simulink model "minseg_M2V3_2017a"  (R2017a)
settings: Solver=FixedStepDiscrete  StartTime=0.0  StopTime=inf  FixedStep=mdl_T_sample  RelTol=1e-3
undefined symbols (not defined in the file or in its folder): ctrl_lqr_K2, ctrl_motorDriver_v_ff_cmd_v_val, ctrl_motorDriver_v_ff_cmd_v_val_norm_dx_max, ctrl_motorDriver_v_ff_cmd_v_val_norm_dx_min, ctrl_motorDriver_v_output_max, ctrl_motorDriver_v_output_min, ctrl_motorDriver_v_pid_cmd_thetaDot_val, ctrl_motorDriver_v_pid_cmd_thetaDot_val_norm_dx_max, ctrl_motorDriver_v_pid_cmd_thetaDot_val_norm_dx_min, ctrl_motorDriver_v_pid_int_maxVal, ctrl_motorDriver_v_pid_int_minVal, ctrl_motorDriver_v_pid_k_d, ctrl_motorDriver_v_pid_k_i, ctrl_motorDriver_v_pid_k_p, ctrl_motorDriver_v_rts_ss_k_A, ctrl_motorDriver_v_rts_ss_k_B, ctrl_motorDriver_v_rts_ss_k_C, ctrl_motorDriver_v_rts_ss_k_D, ctrl_motorDriver_v_rts_ss_stateIC, ctrl_motorDriver_v_sfr_cmd_p_x_f, ctrl_motorDriver_v_sfr_cmd_p_x_mag, ctrl_motorDriver_v_sfr_cmd_p_y_f, ctrl_motorDriver_v_sfr_cmd_p_y_mag, ctrl_motorDriver_v_sfr_K, ctrl_motorDriver_v_sfr_K_plant, ctrl_motorDriver_v_sfr_K_rts, ctrl_motorDriver_v_T_cmd, ctrl_motorDriver_v_T_init, DiscIntNeverNeededParam, gyro_bias, io_srl_read_rateTransition_initialCondition, k_intmax_uint8, mdl_T_sample, mtr_encoder_filter_z_ss_A, mtr_encoder_filter_z_ss_B, mtr_encoder_filter_z_ss_C, mtr_encoder_filter_z_ss_D, plant, plant_accel_k_digital2analog, plant_body_l_c, plant_body_l_w, plant_gyro_encoder_filter_z_den, plant_gyro_encoder_filter_z_num, plant_gyro_filter_z_den, plant_gyro_filter_z_num, plant_gyro_k_digital2analog, plant_linear_ss_stateIC, plant_linear_ss_t_A, plant_linear_ss_t_B, plant_linear_ss_t_C, plant_linear_ss_t_D, plant_mtr_encoder_count2wheelRad, plant_mtr_encoder_filter_z_den, plant_mtr_encoder_filter_z_num, plant_pSupply_v, plant_supply_v, plant_T_init, plant_wheel_r
undefined symbols (not defined in the file): ctrl_lqr_addlDyn_A_discrete, ctrl_lqr_addlDyn_B_discrete, ctrl_lqr_addlDyn_C_discrete, ctrl_lqr_addlDyn_D_discrete, ctrl_lqr_addlDyn_k_antiWindup, ctrl_lqr_addlDyn_stateIC, plant_gyro_bias_movingAverage_n_pts, plant_linear_A_continuous, plant_linear_B_continuous, plant_linear_C_continuous, plant_linear_D_continuous, plant_linear_stateIC
libraries: svdutilitieslib x135, simulink x57, arduinolib x15, MinSegLibrary_M2V3 x3, dspindex x3, RASPlib x2
(part 2 of 6)

== system minseg_M2V3_2017a/Controller [v.motorDriver]/Controller and Enable/Controller/State Feedback Regulation with Reference Tracking System ==
  userIO.read.controller.command : Inport
  plant.state : Inport  Port=2
  Add : Sum  Inputs=-+
  Add1 : Sum  Inputs=--
  Additional Dynamics for Reference Tracking System [Discrete State-Space] : DiscreteStateSpace  A=ctrl_motorDriver_v_rts_ss_k_A  B=ctrl_motorDriver_v_rts_ss_k_B  C=ctrl_motorDriver_v_rts_ss_k_C  D=ctrl_motorDriver_v_rts_ss_k_D  X0=ctrl_motorDriver_v_rts_ss_stateIC  SampleTime=-1
  Gain : Gain  Gain=ctrl_motorDriver_v_sfr_K_plant  Multiplication=Matrix(K*u)
      settings: AttributesFormatString=%<Gain>
  Gain1 : Gain  Gain=ctrl_motorDriver_v_sfr_K_rts  Multiplication=Matrix(K*u)
      settings: AttributesFormatString=%<Gain>
  bus2mux [Command: Reference Tracking System] : Subsystem
  bus2mux [State: Plant] : Subsystem
  bus2mux [State: Reference Tracking System] : Subsystem
  mux2bus [Error: Reference Tracking System] : Subsystem
  output : Outport
  error : Outport  Port=2
  wires:
  bus2mux [State: Reference Tracking System]/1(mux) -> Add/2  "state"
  [KpXp] -> Add1/1  "plant"
  Add/1 -> mux2bus [Error: Reference Tracking System]/1(mux), Additional Dynamics for Reference Tracking System [Discrete State-Space]/1  "error"
  bus2mux [State: Plant]/1(mux) -> Gain/1  "state"
  [plant_state] -> bus2mux [State: Plant]/1(bus)
  plant.state/1 -> [plant_state]
  Additional Dynamics for Reference Tracking System [Discrete State-Space]/1 -> Gain1/1
  Gain1/1 -> Add1/2  "referenceTrackingSystem"
  bus2mux [Command: Reference Tracking System]/1(mux) -> Add/1  "reference"
  Add1/1 -> output/1
  userIO.read.controller.command/1 -> bus2mux [Command: Reference Tracking System]/1(bus)
  Gain/1 -> [KpXp]
  [plant_state] -> bus2mux [State: Reference Tracking System]/1(bus)
  mux2bus [Error: Reference Tracking System]/1(bus) -> error/1

== system minseg_M2V3_2017a/Controller [v.motorDriver]/Saturation/Left-Connected Motor/Saturation flag ==
  u.max : Inport
  u.raw : Inport  Port=2
  u.min : Inport  Port=3
  Add : Sum
  Data Type Conversion : DataTypeConversion  OutDataTypeStr=uint8
  Data Type Conversion1 : DataTypeConversion  OutDataTypeStr=uint8
  Gain : Gain  Gain=uint8(2)  OutDataTypeStr=uint8
      settings: AttributesFormatString=%<Gain>
  Gain1 : Gain  Gain=uint8(1)  OutDataTypeStr=uint8
      settings: AttributesFormatString=%<Gain>
  Relational Operator : RelationalOperator  OutDataTypeStr=boolean  RndMeth=Nearest
  Relational Operator1 : RelationalOperator  Operator=<=  OutDataTypeStr=boolean  RndMeth=Nearest
  x.saturating : Outport
  wires:
  u.raw/1 -> [u_raw]
  [u_raw] -> Relational Operator/1
  u.max/1 -> Relational Operator/2
  [u_raw] -> Relational Operator1/1
  u.min/1 -> Relational Operator1/2
  Add/1 -> x.saturating/1  "x.saturating"
  Relational Operator1/1 -> Data Type Conversion1/1  "x.lowerSaturating"
  Relational Operator/1 -> Data Type Conversion/1  "x.upperSaturating"
  Data Type Conversion/1 -> Gain/1
  Data Type Conversion1/1 -> Gain1/1
  Gain/1 -> Add/1
  Gain1/1 -> Add/2

== system minseg_M2V3_2017a/Controller [v.motorDriver]/Saturation/Middle-Connected Motor/Saturation flag ==
  u.max : Inport
  u.raw : Inport  Port=2
  u.min : Inport  Port=3
  Add : Sum
  Data Type Conversion : DataTypeConversion  OutDataTypeStr=uint8
  Data Type Conversion1 : DataTypeConversion  OutDataTypeStr=uint8
  Gain : Gain  Gain=uint8(2)  OutDataTypeStr=uint8
      settings: AttributesFormatString=%<Gain>
  Gain1 : Gain  Gain=uint8(1)  OutDataTypeStr=uint8
      settings: AttributesFormatString=%<Gain>
  Relational Operator : RelationalOperator  OutDataTypeStr=boolean  RndMeth=Nearest
  Relational Operator1 : RelationalOperator  Operator=<=  OutDataTypeStr=boolean  RndMeth=Nearest
  x.saturating : Outport
  wires:
  Gain1/1 -> Add/2
  Gain/1 -> Add/1
  Data Type Conversion1/1 -> Gain1/1
  Data Type Conversion/1 -> Gain/1
  Relational Operator/1 -> Data Type Conversion/1  "x.upperSaturating"
  Relational Operator1/1 -> Data Type Conversion1/1  "x.lowerSaturating"
  Add/1 -> x.saturating/1  "x.saturating"
  u.min/1 -> Relational Operator1/2
  [u_raw] -> Relational Operator1/1
  u.max/1 -> Relational Operator/2
  [u_raw] -> Relational Operator/1
  u.raw/1 -> [u_raw]

== system minseg_M2V3_2017a/Plant/Hardware/Analog to Digital Conversion/Motor Driver ==
  left.voltage.command : Inport
  middle.voltage.command : Inport  Port=2
  Bus Creator : BusCreator  Inputs=2
  Bus Creator1 : BusCreator  Inputs=2
  Bus Creator{2..4,6,8..9} (6 alike) : BusCreator  Inputs=1
  Left-Connected : Subsystem
  Middle-Connected : Subsystem
  left : Outport
  middle : Outport  Port=2
  wires:
  Bus Creator1/1 -> Bus Creator4/1  "digital"
  Middle-Connected/1(voltage.command.digital.positive) -> Bus Creator1/1  "positive [V]"
  Middle-Connected/2(voltage.command.digital.negative) -> Bus Creator1/2  "negative [V]"
  Bus Creator2/1 -> Bus Creator3/1  "voltage"
  Bus Creator3/1 -> middle/1
  Bus Creator4/1 -> Bus Creator2/1  "command"
  Bus Creator9/1 -> Bus Creator6/1  "command"
  Bus Creator8/1 -> left/1
  middle.voltage.command/1 -> Middle-Connected/1(voltage.command.analog)
  left.voltage.command/1 -> Left-Connected/1(voltage.command.analog)
  Bus Creator6/1 -> Bus Creator8/1  "voltage"
  Left-Connected/2(voltage.command.digital.negative) -> Bus Creator/2  "negative [V]"
  Left-Connected/1(voltage.command.digital.positive) -> Bus Creator/1  "positive [V]"
  Bus Creator/1 -> Bus Creator9/1  "digital"

== system minseg_M2V3_2017a/Plant/Hardware/Arduino Pin IO/Digital Inputs (Reads from Pins) ==
  Accelerometer soMPU6050 : MATLABSystem  System=soMPU6050Accel  SimulateUsing=Code generation
      mask Type: soMPU6050Accel
      mask Display:
      | disp('soMPU6050Accel');
      | port_label('output',1,'xaccel');
      | port_label('output',2,'yaccel');
      | port_label('output',3,'zaccel');
  Bus Creator{1..5,7..8,10..13,16..17} (13 alike) : BusCreator  Inputs=1
  Bus Creator14 : BusCreator  Inputs=2
  Bus Creator15 : BusCreator  Inputs=3
  Bus Creator6 : BusCreator  Inputs=3
  Bus Creator9 : BusCreator  Inputs=3
  Encoder M2V3 - Left Connected - Pins 19,18 : MinSegLibrary_M2V3/M2V3 Left Connector 18, 19  Encoder=1  PinA=19  PinB=18  PWMFSelect=3  PWMTimer=-1
      settings: SourceProductName=Rensselaer Arduino Support Package
  "Encoder M2V3 - Middle Connected - Pins 62, 15" : MinSegLibrary_M2V3/M2V3 Middle Connector 15, 62  Encoder=3  PinA=15  PinB=62  PWMFSelect=3  PWMTimer=-1
      settings: SourceProductName=Rensselaer Arduino Support Package
  Gyroscope soMPU6050 : RASPlib/Gyroscope  DLPFmode=plant_gyro_dlpf_mode
      settings: AttributesFormatString=DLPF mode: %<DLPFmode>  SourceProductName=Rensselaer Arduino Support Package
  Magnetometer : MATLABSystem  System=soHMC5883L  SimulateUsing=Code generation
      mask Type: soHMC5883L
      mask Display:
      | disp('soHMC5883L');
      | port_label('output',1,'xmag');
      | port_label('output',2,'ymag');
      | port_label('output',3,'zmag');
  Pushbutton - Pin A3 : MinSegLibrary_M2V3/User Pushbutton A3  Pin=3
      settings: SourceProductName=Rensselaer Arduino Support Package
  Temperature Sensor (Unspecified) : RASPlib/Temperature  SimulateUsing=Code generation
      settings: SourceProductName=Rensselaer Arduino Support Package
  gyroscope : Outport
  accelerometer : Outport  Port=2
  motorEncoder : Outport  Port=3
  magnetometer : Outport  Port=4
  pushbutton : Outport  Port=5
  tempometer : Outport  Port=6
  wires:
  Bus Creator5/1 -> Bus Creator9/1  "x"
  Bus Creator11/1 -> Bus Creator9/3  "z"
  Encoder M2V3 - Left Connected - Pins 19,18/1 -> Bus Creator13/1  "digital [-]"
  Bus Creator2/1 -> Bus Creator14/2  "middle"
  Bus Creator10/1 -> Bus Creator9/2  "y"
  "Encoder M2V3 - Middle Connected - Pins 62, 15"/1 -> Bus Creator2/1  "digital [-]"
  Accelerometer soMPU6050/3 -> Bus Creator11/1  "digital [-]"
  Accelerometer soMPU6050/1 -> Bus Creator5/1  "digital [-]"
  Accelerometer soMPU6050/2 -> Bus Creator10/1  "digital [-]"
  Bus Creator9/1 -> accelerometer/1
  Bus Creator14/1 -> motorEncoder/1
  Bus Creator13/1 -> Bus Creator14/1  "left"
  Bus Creator3/1 -> Bus Creator6/1  "x"
  Gyroscope soMPU6050/2 -> Bus Creator7/1  "digital [-]"
  Bus Creator6/1 -> gyroscope/1
  Gyroscope soMPU6050/3 -> Bus Creator8/1  "digital [-]"
  Bus Creator7/1 -> Bus Creator6/2  "y"
  Gyroscope soMPU6050/1 -> Bus Creator3/1  "digital [-]"
  Bus Creator8/1 -> Bus Creator6/3  "z"
  Bus Creator15/1 -> magnetometer/1
  Magnetometer/2 -> Bus Creator1/1  "digital [-]"
  Magnetometer/1 -> Bus Creator12/1  "digital [-]"
  Magnetometer/3 -> Bus Creator4/1  "digital [-]"
  Bus Creator1/1 -> Bus Creator15/2  "y"
  Bus Creator4/1 -> Bus Creator15/3  "z"
  Bus Creator12/1 -> Bus Creator15/1  "x"
  Pushbutton - Pin A3/1 -> Bus Creator16/1  "digital [-]"
  Bus Creator16/1 -> pushbutton/1
  Temperature Sensor (Unspecified)/1 -> Bus Creator17/1  "digital [-]"
  Bus Creator17/1 -> tempometer/1

== system minseg_M2V3_2017a/Plant/Hardware/Arduino Pin IO/Digital Outputs (Writes to Pins) ==
  motorDriver.left.voltage.command.digital.positive : Inport
  motorDriver.left.voltage.command.digital.negative : Inport  Port=2
  motorDriver.middle.voltage.command.digital.positive : Inport  Port=3
  motorDriver.middle.voltage.command.digital.negative : Inport  Port=4
  Motor : Subsystem
  wires:
  motorDriver.left.voltage.command.digital.positive/1 -> Motor/1(motor.left.voltage.command.digital.positive)
  motorDriver.left.voltage.command.digital.negative/1 -> Motor/2(motor.left.voltage.command.digital.negative)
  motorDriver.middle.voltage.command.digital.positive/1 -> Motor/3(motor.middle.voltage.command.digital.positive)
  motorDriver.middle.voltage.command.digital.negative/1 -> Motor/4(motor.middle.voltage.command.digital.negative)

== system minseg_M2V3_2017a/Plant/Hardware/Calculations/Body Angular Position (phi) ==
  gyroscope.x : Inport
  gyroscope.y : Inport  Port=2
  gyroscope.z : Inport  Port=3
  accelerometer.x : Inport  Port=4
  accelerometer.y : Inport  Port=5
  accelerometer.z : Inport  Port=6
  wheel.angularPosition.global.left : Inport  Port=7
  wheel.angularPosition.global.middle : Inport  Port=8
  clock.timedEvent.plant.x_initialization : Inport  Port=9
  Bus Creator : BusCreator  Inputs=2
  Bus Creator1 : BusCreator  Inputs=2
  Bus Creator2 : BusCreator  Inputs=2
  X (Pitch) : Subsystem  Variant=on  VariantControl=Variant1
  Y (Yaw) : Subsystem  Variant=on  VariantControl=Variant1
  Z (Roll) : Subsystem  Variant=on  VariantControl=Variant1
  x : Outport
  y : Outport  Port=2
  z : Outport  Port=3
  wires:
  Bus Creator1/1 -> y/1
  Bus Creator/1 -> x/1
  Y (Yaw)/1(" position.y") -> Bus Creator1/1  "position [rad]"
  X (Pitch)/1(" position.x") -> Bus Creator/1  "position [rad]"
  X (Pitch)/2(velocity.x) -> Bus Creator/2  "velocity [rad/s]"
  Z (Roll)/1(position.z) -> Bus Creator2/1  "position [rad]"
  Bus Creator2/1 -> z/1
  gyroscope.x/1 -> X (Pitch)/1(gyroscope.x)
  gyroscope.y/1 -> Y (Yaw)/1(gyroscope.y)
  gyroscope.z/1 -> Z (Roll)/1(gyroscope.z)
  wheel.angularPosition.global.left/1 -> Y (Yaw)/2(wheel.angularPosition.global.left)
  wheel.angularPosition.global.middle/1 -> Y (Yaw)/3(wheel.angularPosition.global.middle)
  accelerometer.y/1 -> [accel_y]
  [accel_y] -> X (Pitch)/2(accelerometer.y)
  accelerometer.z/1 -> [accel_z]
  [accel_z] -> X (Pitch)/3(accelerometer.z)
  Y (Yaw)/2(velocity.y) -> Bus Creator1/2  "velocity [rad/s]"
  Z (Roll)/2(velocity.z) -> Bus Creator2/2  "velocity [rad/s]"
  [accel_y] -> Z (Roll)/3(accelerometer.y)
  [accel_z] -> Z (Roll)/4(accelerometer.z)
  accelerometer.x/1 -> Z (Roll)/2(accelerometer.x)
  clock.timedEvent.plant.x_initialization/1 -> [x_init]
  [x_init] -> X (Pitch)/4(clock.timedEvent.plant.x_initialization)
  [x_init] -> Y (Yaw)/4(clock.timedEvent.plant.x_initialization)
  [x_init] -> Z (Roll)/5(clock.timedEvent.plant.x_initialization)

== system minseg_M2V3_2017a/Plant/Hardware/Calculations/Linear Position (p) ==
  wheel.angularVelocity.global : Inport
  body.angularPosition.x (pitch) : Inport  Port=2
  body.angularPosition.y (yaw) : Inport  Port=3
  Body : Subsystem
  Bus Creator1 : BusCreator  Inputs=3
  Bus Creator4 : BusCreator  Inputs=3
  Bus Selector1 : BusSelector  OutputSignals=center.x.position [m],center.y.position [m],center.z.position [m]
  Wheel : Subsystem
  wheel : Outport
  body : Outport  Port=2
  wires:
  [p_wheel] -> Bus Selector1/1
  Bus Creator4/1 -> [p_wheel], wheel/1
  Wheel/3(center) -> Bus Creator4/3  "center"
  wheel.angularVelocity.global/1 -> Wheel/1(wheel.angularVelocity.global)
  Wheel/2(middle) -> Bus Creator4/2  "middle"
  Wheel/1(left) -> Bus Creator4/1  "left"
  Bus Selector1/2 -> Body/2(p.center.y)  "<position [m]>"
  Bus Selector1/1 -> Body/1(p.center.x)  "<position [m]>"
  Bus Selector1/3 -> Body/3(p.center.z)  "<position [m]>"
  body.angularPosition.y (yaw)/1 -> [yaw]
  [yaw] -> Wheel/2(body.angularPosition.y (yaw))
  body.angularPosition.x (pitch)/1 -> Body/4(body.angularPosition.x (pitch))
  [yaw] -> Body/5(body.angularPosition.y (yaw))
  Bus Creator1/1 -> body/1
  Body/1(x) -> Bus Creator1/1  "x"
  Body/2(y) -> Bus Creator1/2  "y"
  Body/3(z) -> Bus Creator1/3  "z"

== system minseg_M2V3_2017a/Plant/Hardware/Calculations/Wheel Angular Position (theta) ==
  motorEncoder.left : Inport
  motorEncoder.middle : Inport  Port=2
  body.angularPosition.x (pitch) : Inport  Port=3
  Bus Creator1 : BusCreator  Inputs=3
  Bus Creator4 : BusCreator  Inputs=3
  Bus Selector1 : BusSelector  OutputSignals=left.position [rad],middle.position [rad]
  Reference Point: Body : Subsystem
  Reference Point: Earth : Subsystem
  body : Outport
  global : Outport  Port=2
  wires:
  motorEncoder.left/1 -> Reference Point: Body/1(motorEncoder.left)
  motorEncoder.middle/1 -> Reference Point: Body/2(motorEncoder.middle)
  Bus Creator4/1 -> [theta_body], body/1
  Bus Creator1/1 -> global/1
  Reference Point: Body/2(middle) -> Bus Creator4/2  "middle"
  Reference Point: Body/1(left) -> Bus Creator4/1  "left"
  Reference Point: Body/3(average) -> Bus Creator4/3  "average"
  [theta_body] -> Bus Selector1/1
  Reference Point: Earth/1(left) -> Bus Creator1/1  "left"
  Reference Point: Earth/2(middle) -> Bus Creator1/2  "middle"
  Reference Point: Earth/3(average) -> Bus Creator1/3  "average"
  Bus Selector1/1 -> Reference Point: Earth/1(wheel.left.angularPosition.body)  "<position [rad]>"
  Bus Selector1/2 -> Reference Point: Earth/2(wheel.middle.angularPosition.body)  "<position [rad]>"
  body.angularPosition.x (pitch)/1 -> Reference Point: Earth/3(body.angularPosition.x (pitch))

== system minseg_M2V3_2017a/Plant/Hardware/Digital to Analog Conversion/Accelerometer ==
  x.digital : Inport
  y.digital : Inport  Port=2
  z.digital : Inport  Port=3
  Data Type Conversion1 : DataTypeConversion  OutDataTypeStr=double
  Data Type Conversion2 : DataTypeConversion  OutDataTypeStr=double
  Data Type Conversion3 : DataTypeConversion  OutDataTypeStr=double
  Gain1 : Gain  Gain=plant_accel_k_digital2analog
      settings: AttributesFormatString=%<Gain>
  Gain2 : Gain  Gain=plant_accel_k_digital2analog
      settings: AttributesFormatString=%<Gain>
  Gain3 : Gain  Gain=plant_accel_k_digital2analog
      settings: AttributesFormatString=%<Gain>
  x.analog : Outport
  y.analog : Outport  Port=2
  z.analog : Outport  Port=3
  wires:
  z.digital/1 -> Data Type Conversion3/1
  y.digital/1 -> Data Type Conversion2/1
  Gain2/1 -> y.analog/1
  Gain3/1 -> z.analog/1
  Gain1/1 -> x.analog/1
  Data Type Conversion1/1 -> Gain1/1
  x.digital/1 -> Data Type Conversion1/1
  Data Type Conversion2/1 -> Gain2/1
  Data Type Conversion3/1 -> Gain3/1

== system minseg_M2V3_2017a/Plant/Hardware/Digital to Analog Conversion/Gyroscope ==
  x.digital : Inport
  y.digital : Inport  Port=2
  z.digital : Inport  Port=3
  clock.timedEvent.plant.x_initialization : Inport  Port=4
  x : Subsystem
  y : Subsystem
  z : Subsystem
  x.analog : Outport
  y.analog : Outport  Port=2
  z.analog : Outport  Port=3
  wires:
  x/1(analog) -> x.analog/1
  x.digital/1 -> x/1(digital)
  [x_init] -> x/2(clock.timedEvent.plant.x_initialization)
  clock.timedEvent.plant.x_initialization/1 -> [x_init]
  [x_init] -> y/2(clock.timedEvent.model.initialization)
  y.digital/1 -> y/1(digital)
  y/1(analog) -> y.analog/1
  [x_init] -> z/2(clock.timedEvent.model.initialization)
  z.digital/1 -> z/1(digital)
  z/1(analog) -> z.analog/1

== system minseg_M2V3_2017a/Plant/Hardware/Digital to Analog Conversion/Magnetometer (Incomplete) ==
  x.digital : Inport
  y.digital : Inport  Port=2
  z.digital : Inport  Port=3
  Data Type Conversion1 : DataTypeConversion  OutDataTypeStr=double
  Data Type Conversion2 : DataTypeConversion  OutDataTypeStr=double
  Data Type Conversion3 : DataTypeConversion  OutDataTypeStr=double
  x.analog : Outport
  y.analog : Outport  Port=2
  z.analog : Outport  Port=3
  wires:
  y.digital/1 -> Data Type Conversion2/1
  z.digital/1 -> Data Type Conversion3/1
  x.digital/1 -> Data Type Conversion1/1
  Data Type Conversion1/1 -> x.analog/1
  Data Type Conversion2/1 -> y.analog/1
  Data Type Conversion3/1 -> z.analog/1

== system minseg_M2V3_2017a/Plant/Hardware/Digital to Analog Conversion/Motor Encoder ==
  left.digital : Inport
  middle.digital : Inport  Port=2
  Data Type Conversion : DataTypeConversion  OutDataTypeStr=double
      settings: AttributesFormatString=saturateOverflow(%<SaturateOnIntegerOverflow>)
  Data Type Conversion1 : DataTypeConversion  OutDataTypeStr=double
      settings: AttributesFormatString=saturateOverflow(%<SaturateOnIntegerOverflow>)
  Gain3 : Gain  Gain=plant_mtr_encoder_count2wheelRad
      settings: AttributesFormatString=%<Gain>
  Gain4 : Gain  Gain=plant_mtr_encoder_count2wheelRad
      settings: AttributesFormatString=%<Gain>
  left.analog : Outport
  middle.analog : Outport  Port=2
  wires:
  middle.digital/1 -> Data Type Conversion1/1
  left.digital/1 -> Data Type Conversion/1
  Data Type Conversion/1 -> Gain4/1
  Data Type Conversion1/1 -> Gain3/1
  Gain4/1 -> left.analog/1
  Gain3/1 -> middle.analog/1

== system minseg_M2V3_2017a/Plant/Hardware/Digital to Analog Conversion/Pushbutton (Incomplete) ==
  digital : Inport
  Data Type Conversion1 : DataTypeConversion  OutDataTypeStr=double
  analog : Outport
  wires:
  digital/1 -> Data Type Conversion1/1
  Data Type Conversion1/1 -> analog/1

== system minseg_M2V3_2017a/Plant/Hardware/Digital to Analog Conversion/Tempometer (Incomplete) ==
  digital : Inport
  Data Type Conversion1 : DataTypeConversion  OutDataTypeStr=double
  analog : Outport
  wires:
  digital/1 -> Data Type Conversion1/1
  Data Type Conversion1/1 -> analog/1

== system minseg_M2V3_2017a/Plant/Hardware-Equivalent Linear Dynamics/Calculation/Linear Position (p) ==
  wheel.angularVelocity.global : Inport
  body.angularPosition.x (pitch) : Inport  Port=2
  body.angularPosition.y (yaw) : Inport  Port=3
  Body : Subsystem
  Bus Creator1 : BusCreator  Inputs=3
  Bus Creator4 : BusCreator  Inputs=3
  Bus Selector1 : BusSelector  OutputSignals=center.x.position [m],center.y.position [m],center.z.position [m]
  Wheel : Subsystem
  wheel : Outport
  body : Outport  Port=2
  wires:
  [p_wheel] -> Bus Selector1/1
  Bus Creator4/1 -> [p_wheel], wheel/1
  Wheel/3(center) -> Bus Creator4/3  "center"
  wheel.angularVelocity.global/1 -> Wheel/1(wheel.angularVelocity.global)
  Wheel/2(middle) -> Bus Creator4/2  "middle"
  Wheel/1(left) -> Bus Creator4/1  "left"
  Bus Selector1/2 -> Body/2(p.center.y)  "<position [m]>"
  Bus Selector1/1 -> Body/1(p.center.x)  "<position [m]>"
  Bus Selector1/3 -> Body/3(p.center.z)  "<position [m]>"
  body.angularPosition.y (yaw)/1 -> [yaw]
  [yaw] -> Wheel/2(body.angularPosition.y (yaw))
  body.angularPosition.x (pitch)/1 -> Body/4(body.angularPosition.x (pitch))
  [yaw] -> Body/5(body.angularPosition.y (yaw))
  Bus Creator1/1 -> body/1
  Body/1(x) -> Bus Creator1/1  "x"
  Body/2(y) -> Bus Creator1/2  "y"
  Body/3(z) -> Bus Creator1/3  "z"

== system minseg_M2V3_2017a/Plant/Hardware-Equivalent Linear Dynamics/Calculation/Wheel Angular Position (theta) ==
  wheel.angularPosition.global.average : Inport
  wheel.angularVelocity.global.average : Inport  Port=2
  body.angularPosition.x (pitch) : Inport  Port=3
  body.angularPosition.y (yaw) : Inport  Port=4
  Bus Creator1 : BusCreator  Inputs=3
  Bus Creator4 : BusCreator  Inputs=3
  Bus Selector1 : BusSelector  OutputSignals=left.position [rad],middle.position [rad]
  Reference Point: Body : Subsystem
  Reference Point: Earth : Subsystem
  body : Outport
  global : Outport  Port=2
  wires:
  Bus Creator4/1 -> body/1
  Reference Point: Body/2(middle) -> Bus Creator4/2  "middle"
  Reference Point: Body/1(left) -> Bus Creator4/1  "left"
  Reference Point: Body/3(average) -> Bus Creator4/3  "average"
  Reference Point: Earth/1(left) -> Bus Creator1/1  "left"
  Reference Point: Earth/2(middle) -> Bus Creator1/2  "middle"
  Reference Point: Earth/3(average) -> Bus Creator1/3  "average"
  Bus Creator1/1 -> [theta_global], global/1
  [theta_global] -> Bus Selector1/1
  Bus Selector1/1 -> Reference Point: Body/1(wheel.angularPosition.global.left)  "<position [rad]>"
  Bus Selector1/2 -> Reference Point: Body/2(wheel.angularPosition.global.middle)  "<position [rad]>"
  wheel.angularVelocity.global.average/1 -> Reference Point: Earth/2(wheel.angularVelocity.global.average)
  wheel.angularPosition.global.average/1 -> Reference Point: Earth/1(wheel.angularPosition.global.average)
  body.angularPosition.y (yaw)/1 -> Reference Point: Earth/3(body.angularPosition.y (yaw))
  body.angularPosition.x (pitch)/1 -> Reference Point: Body/3(body.angularPosition.x (pitch))

== system minseg_M2V3_2017a/User IO/Reads (From PC)/Controller/Feed-Forward ==
  note: Make rate limitiing 0-centric
  Bus Creator1 : BusCreator  Inputs=1
  Bus Creator2 : BusCreator  Inputs=2
  Bus Creator3 : BusCreator  Inputs=1
  Gain1 : Gain  Gain=ctrl_motorDriver_v_ff_cmd_v_val
      settings: AttributesFormatString=%<Gain>
  Rate Limiter 1 : RateLimiter  RisingSlewLimit=ctrl_motorDriver_v_ff_cmd_v_val_norm_dx_max  FallingSlewLimit=ctrl_motorDriver_v_ff_cmd_v_val_norm_dx_min  SampleTimeMode=inherited
      settings: AttributesFormatString=|
      | dx_max: %<RisingSlewLimit>
      | dx_min: %<FallingSlewLimit>
  Step 1 : Step  Time=0  SampleTime=mdl_T_sample
      settings: AttributesFormatString=t.start: %<Time>
  command : Outport
  wires:
  Gain1/1 -> Bus Creator1/1, Bus Creator3/1  "motorDriver_v [V]"
  Rate Limiter 1/1 -> Gain1/1
  Bus Creator2/1 -> command/1
  Bus Creator1/1 -> Bus Creator2/2  "middle"
  Bus Creator3/1 -> Bus Creator2/1  "left"
  Step 1/1 -> Rate Limiter 1/1

== system minseg_M2V3_2017a/User IO/Reads (From PC)/Controller/PID ==
  note: Make rate limitiing 0-centric
  Bus Creator1 : BusCreator  Inputs=1
  Bus Creator2 : BusCreator  Inputs=2
  Bus Creator3 : BusCreator  Inputs=1
  Gain1 : Gain  Gain=ctrl_motorDriver_v_pid_cmd_thetaDot_val
      settings: AttributesFormatString=%<Gain>
  Rate Limiter 1 : RateLimiter  RisingSlewLimit=ctrl_motorDriver_v_pid_cmd_thetaDot_val_norm_dx_max  FallingSlewLimit=ctrl_motorDriver_v_pid_cmd_thetaDot_val_norm_dx_min  SampleTimeMode=inherited
      settings: AttributesFormatString=|
      | dx_max: %<RisingSlewLimit>
      | dx_min: %<FallingSlewLimit>
  Step 1 : Step  Time=0  SampleTime=mdl_T_sample
      settings: AttributesFormatString=t.start: %<Time>
  command : Outport
  wires:
  Bus Creator3/1 -> Bus Creator2/1  "left"
  Bus Creator2/1 -> command/1
  Gain1/1 -> Bus Creator3/1, Bus Creator1/1  "theta_global_average_dot [rad/s]"
  Bus Creator1/1 -> Bus Creator2/2  "middle"
  Step 1/1 -> Rate Limiter 1/1
  Rate Limiter 1/1 -> Gain1/1

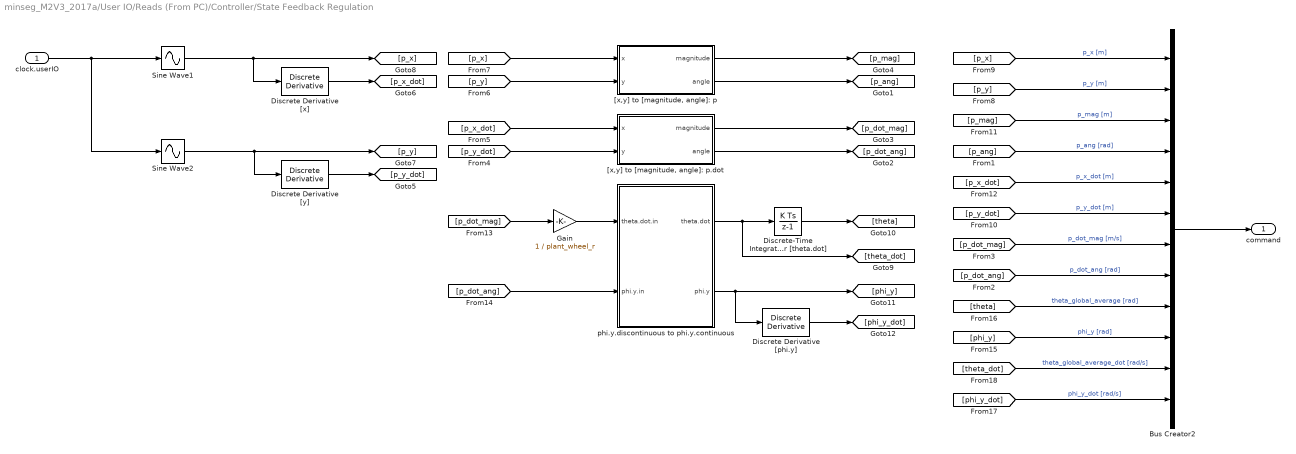
== system minseg_M2V3_2017a/User IO/Reads (From PC)/Controller/State Feedback Regulation ==
  clock.userIO : Inport
  Bus Creator2 : BusCreator  Inputs=12
  Discrete Derivative [phi.y] : simulink/Discrete/Discrete Derivative  gainval=1.0  ICPrevScaledInput=0.0  OutMin=[]  OutMax=[]  OutDataType=fixdt(1, 16)  OutScaling=2^-10  DoSatur=off
  Discrete Derivative [x] : simulink/Discrete/Discrete Derivative  gainval=1.0  ICPrevScaledInput=0.0  OutMin=[]  OutMax=[]  OutDataType=fixdt(1, 16)  OutScaling=2^-10  DoSatur=off
  Discrete Derivative [y] : simulink/Discrete/Discrete Derivative  gainval=1.0  ICPrevScaledInput=0.0  OutMin=[]  OutMax=[]  OutDataType=fixdt(1, 16)  OutScaling=2^-10  DoSatur=off
  Discrete-Time Integrator [theta.dot] : DiscreteIntegrator  InitialConditionSetting=State (most efficient)  SampleTime=-1  ICPrevOutput=DiscIntNeverNeededParam  ICPrevScaledInput=DiscIntNeverNeededParam
  Gain : Gain  Gain=1 / plant_wheel_r
      settings: AttributesFormatString=%<Gain>
  Sine Wave1 : Sin  TimeSource=Use external signal  Amplitude=ctrl_motorDriver_v_sfr_cmd_p_x_mag  Frequency=2 * pi * ctrl_motorDriver_v_sfr_cmd_p_x_f  SampleTime=mdl_T_sample
      settings: AttributesFormatString=|
      | amplitude:
      | %<Amplitude>
      | 
      | angular frequency:
      | %<Frequency>
  Sine Wave2 : Sin  TimeSource=Use external signal  Amplitude=ctrl_motorDriver_v_sfr_cmd_p_y_mag  Frequency=2 * pi * ctrl_motorDriver_v_sfr_cmd_p_y_f  SampleTime=mdl_T_sample
      settings: AttributesFormatString=|
      | amplitude:
      | %<Amplitude>
      | 
      | angular frequency:
      | %<Frequency>
  "[x,y] to [magnitude, angle]: p" : Subsystem
  "[x,y] to [magnitude, angle]: p.dot" : Subsystem
  phi.y.discontinuous to phi.y.continuous : Subsystem
  command : Outport
  wires:
  Bus Creator2/1 -> command/1
  [p_x] -> Bus Creator2/1  "p_x [m]"
  [p_y] -> Bus Creator2/2  "p_y [m]"
  "[x,y] to [magnitude, angle]: p"/1(magnitude) -> [p_mag]
  "[x,y] to [magnitude, angle]: p"/2(angle) -> [p_ang]
  Sine Wave1/1 -> [p_x], Discrete Derivative [x]/1
  "[x,y] to [magnitude, angle]: p.dot"/1(magnitude) -> [p_dot_mag]
  "[x,y] to [magnitude, angle]: p.dot"/2(angle) -> [p_dot_ang]
  Sine Wave2/1 -> Discrete Derivative [y]/1, [p_y]
  Discrete Derivative [y]/1 -> [p_y_dot]
  Discrete Derivative [x]/1 -> [p_x_dot]
  [p_x] -> "[x,y] to [magnitude, angle]: p"/1(x)
  [p_y] -> "[x,y] to [magnitude, angle]: p"/2(y)
  [p_x_dot] -> "[x,y] to [magnitude, angle]: p.dot"/1(x)
  [p_y_dot] -> "[x,y] to [magnitude, angle]: p.dot"/2(y)
  [p_mag] -> Bus Creator2/3  "p_mag [m]"
  [p_ang] -> Bus Creator2/4  "p_ang [rad]"
  [p_x_dot] -> Bus Creator2/5  "p_x_dot [m]"
  [p_y_dot] -> Bus Creator2/6  "p_y_dot [m]"
  [p_dot_mag] -> Bus Creator2/7  "p_dot_mag [m/s]"
  [p_dot_ang] -> Bus Creator2/8  "p_dot_ang [rad]"
  [theta] -> Bus Creator2/9  "theta_global_average [rad]"
  [phi_y] -> Bus Creator2/10  "phi_y [rad]"
  [phi_y_dot] -> Bus Creator2/12  "phi_y_dot [rad/s]"
  [theta_dot] -> Bus Creator2/11  "theta_global_average_dot [rad/s]"
  clock.userIO/1 -> Sine Wave2/1, Sine Wave1/1
  [p_dot_ang] -> phi.y.discontinuous to phi.y.continuous/2(phi.y.in)
  [p_dot_mag] -> Gain/1
  Gain/1 -> phi.y.discontinuous to phi.y.continuous/1(theta.dot.in)
  Discrete-Time Integrator [theta.dot]/1 -> [theta]
  Discrete Derivative [phi.y]/1 -> [phi_y_dot]
  phi.y.discontinuous to phi.y.continuous/1(theta.dot) -> [theta_dot], Discrete-Time Integrator [theta.dot]/1
  phi.y.discontinuous to phi.y.continuous/2(phi.y) -> Discrete Derivative [phi.y]/1, [phi_y]

== system minseg_M2V3_2017a/User IO/Writes (To PC)/Plant: Hardware/Controller: FF ==
  note: There is no need to change the datatype paramter
      | listed in the Byte Pack blocks.
      |
      | It will update automatically based on the datatype parameter
      | listed in the Datatype Conversion Block,
      | through the use of the initialization script.
  systemSignalBus : Inport
  Bus Selector : BusSelector  OutputSignals=clock.time [s],userIO.read.controller.command.left.motorDriver_v [V],userIO.read.controller.command.middle.motorDriver_v [V],plant.hardware.pin.digital.out(ToPin).motorDriver.left.voltage.command.digital.positive [V],plant.hardware.pin.digital.out(ToPin).motorDriver.left.voltage.command.digital.negative [V],plant.hardware.pin.digital.out(ToPin).motorDriver.middle.voltage.command.digital.positive [V],plant.hardware.pin.digital.out(ToPin).motorDriver.middle.voltage.command.digital.negative [V],plant.position.theta.body.left.position [rad],plant.position.theta.body.middle.position [rad],plant.position.phi.x (pitch).position [rad],plant.position.theta.global.average.position [rad],plant.position.phi.y (yaw).position [rad]
  Byte Pack - 01 : svdutilitieslib/Byte Pack  datatypes={'single'}  byteAlign=1  blockPlatform=arduinoert
      settings: AttributesFormatString=%<datatypes>  SourceProductName=Simulink Support Package for Arduino Hardware
  Byte Pack - 02 : svdutilitieslib/Byte Pack  datatypes={'single'}  byteAlign=1  blockPlatform=arduinoert
      settings: AttributesFormatString=%<datatypes>  SourceProductName=Simulink Support Package for Arduino Hardware
  Byte Pack - 03 : svdutilitieslib/Byte Pack  datatypes={'single'}  byteAlign=1  blockPlatform=arduinoert
      settings: AttributesFormatString=%<datatypes>  SourceProductName=Simulink Support Package for Arduino Hardware
  Byte Pack - 04 : svdutilitieslib/Byte Pack  datatypes={'uint8'}  byteAlign=1  blockPlatform=arduinoert
      settings: AttributesFormatString=%<datatypes>  SourceProductName=Simulink Support Package for Arduino Hardware
  Byte Pack - 05 : svdutilitieslib/Byte Pack  datatypes={'uint8'}  byteAlign=1  blockPlatform=arduinoert
      settings: AttributesFormatString=%<datatypes>  SourceProductName=Simulink Support Package for Arduino Hardware
  Byte Pack - 06 : svdutilitieslib/Byte Pack  datatypes={'uint8'}  byteAlign=1  blockPlatform=arduinoert
      settings: AttributesFormatString=%<datatypes>  SourceProductName=Simulink Support Package for Arduino Hardware
  Byte Pack - 07 : svdutilitieslib/Byte Pack  datatypes={'uint8'}  byteAlign=1  blockPlatform=arduinoert
      settings: AttributesFormatString=%<datatypes>  SourceProductName=Simulink Support Package for Arduino Hardware
  Byte Pack - 08 : svdutilitieslib/Byte Pack  datatypes={'single'}  byteAlign=1  blockPlatform=arduinoert
      settings: AttributesFormatString=%<datatypes>  SourceProductName=Simulink Support Package for Arduino Hardware
  Byte Pack - 09 : svdutilitieslib/Byte Pack  datatypes={'single'}  byteAlign=1  blockPlatform=arduinoert
      settings: AttributesFormatString=%<datatypes>  SourceProductName=Simulink Support Package for Arduino Hardware
  Byte Pack - 10 : svdutilitieslib/Byte Pack  datatypes={'single'}  byteAlign=1  blockPlatform=arduinoert
      settings: AttributesFormatString=%<datatypes>  SourceProductName=Simulink Support Package for Arduino Hardware
  Byte Pack - 11 : svdutilitieslib/Byte Pack  datatypes={'single'}  byteAlign=1  blockPlatform=arduinoert
      settings: AttributesFormatString=%<datatypes>  SourceProductName=Simulink Support Package for Arduino Hardware
  Byte Pack - 12 : svdutilitieslib/Byte Pack  datatypes={'single'}  byteAlign=1  blockPlatform=arduinoert
      settings: AttributesFormatString=%<datatypes>  SourceProductName=Simulink Support Package for Arduino Hardware
  Data Type Conversion - 01 : DataTypeConversion  OutDataTypeStr=single
  Data Type Conversion - 02 : DataTypeConversion  OutDataTypeStr=single
  Data Type Conversion - 03 : DataTypeConversion  OutDataTypeStr=single
  Data Type Conversion - 04 : DataTypeConversion  OutDataTypeStr=uint8
  Data Type Conversion - 05 : DataTypeConversion  OutDataTypeStr=uint8
  Data Type Conversion - 06 : DataTypeConversion  OutDataTypeStr=uint8
  Data Type Conversion - 07 : DataTypeConversion  OutDataTypeStr=uint8
  Data Type Conversion - 08 : DataTypeConversion  OutDataTypeStr=single
  Data Type Conversion - 09 : DataTypeConversion  OutDataTypeStr=single
  Data Type Conversion - 10 : DataTypeConversion  OutDataTypeStr=single
  Data Type Conversion - 11 : DataTypeConversion  OutDataTypeStr=single
  Data Type Conversion - 12 : DataTypeConversion  OutDataTypeStr=single
  Mux : Mux  Inputs=12
  Rate Transition : RateTransition  X0=0 %io_srl_read_rateTransition_initialCondition  OutPortSampleTimeMultiple=io_read_rateTransition_decimation  OutPortSampleTime=io_srl_read_rateTransition_T_sample
      settings: AttributesFormatString=|
      | Output sample time: %<OutPortSampleTime>
      | Initial condition: %<X0>
  Serial Transmit : arduinolib/Serial Transmit  portNumber=srl_port  sendmode=write  sendformat=Decimal  floatprecision=2  blockPlatform=arduino
      settings: SourceProductName=Simulink Support Package for Arduino Hardware
  wires:
  Bus Selector/1 -> Data Type Conversion - 01/1  "<time [s]>"
  Mux/1 -> Serial Transmit/1
  Bus Selector/4 -> Data Type Conversion - 04/1  "<positive [V]>"
  Bus Selector/3 -> Data Type Conversion - 03/1  "<motorDriver_v [V]>"
  Byte Pack - 12/1 -> Mux/12
  Byte Pack - 11/1 -> Mux/11
  Data Type Conversion - 11/1 -> Byte Pack - 11/1
  Data Type Conversion - 12/1 -> Byte Pack - 12/1
  Data Type Conversion - 10/1 -> Byte Pack - 10/1
  Data Type Conversion - 09/1 -> Byte Pack - 09/1
  Data Type Conversion - 08/1 -> Byte Pack - 08/1
  Data Type Conversion - 07/1 -> Byte Pack - 07/1
  Data Type Conversion - 06/1 -> Byte Pack - 06/1
  Data Type Conversion - 05/1 -> Byte Pack - 05/1
  Data Type Conversion - 04/1 -> Byte Pack - 04/1
  Data Type Conversion - 03/1 -> Byte Pack - 03/1
  Data Type Conversion - 02/1 -> Byte Pack - 02/1
  Data Type Conversion - 01/1 -> Byte Pack - 01/1
  Byte Pack - 10/1 -> Mux/10
  Byte Pack - 09/1 -> Mux/9
  Bus Selector/2 -> Data Type Conversion - 02/1  "<motorDriver_v [V]>"
  systemSignalBus/1 -> Rate Transition/1
  Byte Pack - 02/1 -> Mux/2
  Byte Pack - 08/1 -> Mux/8
  Byte Pack - 05/1 -> Mux/5
  Byte Pack - 06/1 -> Mux/6
  Byte Pack - 01/1 -> Mux/1
  Byte Pack - 07/1 -> Mux/7
  Byte Pack - 03/1 -> Mux/3
  Byte Pack - 04/1 -> Mux/4
  Bus Selector/5 -> Data Type Conversion - 05/1  "<negative [V]>"
  Bus Selector/6 -> Data Type Conversion - 06/1  "<positive [V]>"
  Bus Selector/7 -> Data Type Conversion - 07/1  "<negative [V]>"
  Bus Selector/8 -> Data Type Conversion - 08/1  "<position [rad]>"
  Bus Selector/9 -> Data Type Conversion - 09/1  "<position [rad]>"
  Rate Transition/1 -> Bus Selector/1
  Bus Selector/12 -> Data Type Conversion - 12/1  "<position [rad]>"
  Bus Selector/10 -> Data Type Conversion - 10/1  "<position [rad]>"
  Bus Selector/11 -> Data Type Conversion - 11/1  "<position [rad]>"

== system minseg_M2V3_2017a/User IO/Writes (To PC)/Plant: Hardware/Controller: PID ==
  "systemSignalBus " : Inport
  MPU6050 Calibration : Subsystem  VariantControl=mdl_sensorCalibration_var
  Standard : Subsystem  VariantControl=(default)

== system minseg_M2V3_2017a/User IO/Writes (To PC)/Plant: Hardware/Controller: SFR ==
  "systemSignalBus " : Inport
  MPU6050 Calibration : Subsystem  VariantControl=mdl_sensorCalibration_var
  Motor Characterization : Subsystem  VariantControl=mdl_motorCharacterization_var
  Standard : Subsystem  VariantControl=(default)

== system minseg_M2V3_2017a/User IO/Writes (To PC)/Plant: Linear Dynamics/Controller: FF ==
  "systemSignalBus " : Inport
  Motor Characterization : Subsystem  VariantControl=mdl_motorCharacterization_var
  Standard : Subsystem  VariantControl=(default)

== system minseg_M2V3_2017a/User IO/Writes (To PC)/Plant: Linear Dynamics/Controller: PID ==
  "systemSignalBus " : Inport
  MPU6050 Calibration : Subsystem  VariantControl=mdl_sensorCalibration_var
  Motor Characterization : Subsystem  VariantControl=mdl_motorCharacterization_var
  Standard : Subsystem  VariantControl=(default)

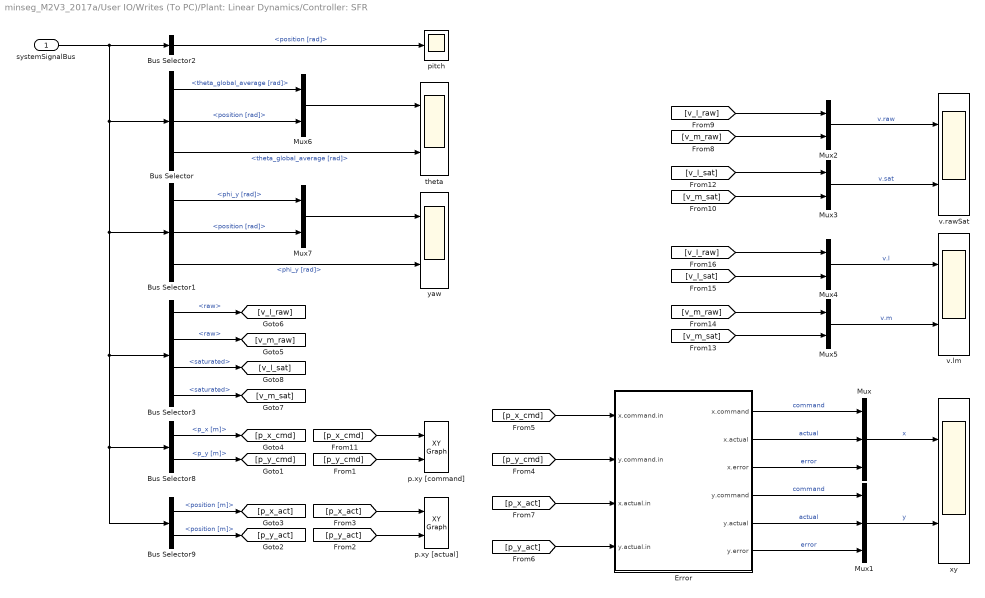
== system minseg_M2V3_2017a/User IO/Writes (To PC)/Plant: Linear Dynamics/Controller: SFR ==
  systemSignalBus : Inport
  Bus Selector : BusSelector  OutputSignals=userIO.read.controller.command.theta_global_average [rad],plant.position.theta.global.average.position [rad],userIO.read.controller.command.theta_global_average [rad]
  Bus Selector1 : BusSelector  OutputSignals=userIO.read.controller.command.phi_y [rad],plant.position.phi.y (yaw).position [rad],controller.v_motorDriver.error.phi_y [rad]
  Bus Selector2 : BusSelector  OutputSignals=plant.position.phi.x (pitch).position [rad]
  Bus Selector3 : BusSelector  OutputSignals=controller.v_motorDriver.output.left.command [V].raw,controller.v_motorDriver.output.middle.command [V].raw,controller.v_motorDriver.output.left.command [V].saturated,controller.v_motorDriver.output.middle.command [V].saturated
  Bus Selector8 : BusSelector  OutputSignals=userIO.read.controller.command.p_x [m],userIO.read.controller.command.p_y [m]
  Bus Selector9 : BusSelector  OutputSignals=plant.position.p.wheel.center.x.position [m],plant.position.p.wheel.center.y.position [m]
  Error : Subsystem
  Mux : Mux  Inputs=3
  Mux1 : Mux  Inputs=3
  Mux{2..7} (6 alike) : Mux  Inputs=2
  p.xy [actual] : simulink/Sinks/XY Graph  xmin=-1  xmax=+1  ymin=-1  ymax=+1  st=-1
  p.xy [command] : simulink/Sinks/XY Graph  xmin=-1  xmax=+1  ymin=-1  ymax=+1  st=-1
  pitch : Scope
  theta : Scope  NumInputPorts=2
  v.lm : Scope  NumInputPorts=2
  v.rawSat : Scope  NumInputPorts=2
  xy : Scope  NumInputPorts=2
  yaw : Scope  NumInputPorts=2
  wires:
  Error/1(x.command) -> Mux/1  "command"
  Error/2(x.actual) -> Mux/2  "actual"
  Error/3(x.error) -> Mux/3  "error"
  Error/4(y.command) -> Mux1/1  "command"
  systemSignalBus/1 -> Bus Selector9/1, Bus Selector8/1, Bus Selector3/1, Bus Selector1/1, Bus Selector/1, Bus Selector2/1
  Bus Selector2/1 -> pitch/1  "<position [rad]>"
  Bus Selector1/3 -> yaw/2  "<phi_y [rad]>"
  Bus Selector/3 -> theta/2  "<theta_global_average [rad]>"
  Error/5(y.actual) -> Mux1/2  "actual"
  Error/6(y.error) -> Mux1/3  "error"
  Mux/1 -> xy/1  "x"
  Mux1/1 -> xy/2  "y"
  Bus Selector8/1 -> [p_x_cmd]  "<p_x [m]>"
  Bus Selector8/2 -> [p_y_cmd]  "<p_y [m]>"
  Bus Selector9/1 -> [p_x_act]  "<position [m]>"
  Bus Selector9/2 -> [p_y_act]  "<position [m]>"
  [p_x_cmd] -> p.xy [command]/1
  [p_y_cmd] -> p.xy [command]/2
  [p_x_act] -> p.xy [actual]/1
  [p_y_act] -> p.xy [actual]/2
  [p_x_cmd] -> Error/1(x.command.in)
  [p_x_act] -> Error/3(x.actual.in)
  [p_y_cmd] -> Error/2(y.command.in)
  [p_y_act] -> Error/4(y.actual.in)
  Bus Selector3/1 -> [v_l_raw]  "<raw>"
  Bus Selector3/2 -> [v_m_raw]  "<raw>"
  Bus Selector3/4 -> [v_m_sat]  "<saturated>"
  Bus Selector3/3 -> [v_l_sat]  "<saturated>"
  [v_m_raw] -> Mux2/2
  [v_l_raw] -> Mux2/1
  Mux2/1 -> v.rawSat/1  "v.raw"
  [v_l_sat] -> Mux3/1
  [v_m_sat] -> Mux3/2
  Mux3/1 -> v.rawSat/2  "v.sat"
  Mux5/1 -> v.lm/2  "v.m"
  [v_m_sat] -> Mux5/2
  [v_m_raw] -> Mux5/1
  Mux4/1 -> v.lm/1  "v.l"
  [v_l_raw] -> Mux4/1
  [v_l_sat] -> Mux4/2
  Bus Selector/1 -> Mux6/1  "<theta_global_average [rad]>"
  Bus Selector/2 -> Mux6/2  "<position [rad]>"
  Mux6/1 -> theta/1
  Bus Selector1/1 -> Mux7/1  "<phi_y [rad]>"
  Bus Selector1/2 -> Mux7/2  "<position [rad]>"
  Mux7/1 -> yaw/1

== system minseg_M2V3_2017a/User IO/Writes (To PC)/Plant: Nonlinear Dynamics/Controller: FF ==
  "systemSignalBus " : Inport
  Standard : Subsystem  VariantControl=(default)

== system minseg_M2V3_2017a/User IO/Writes (To PC)/Plant: Nonlinear Dynamics/Controller: PID ==
  "systemSignalBus " : Inport
  Standard : Subsystem  VariantControl=(default)

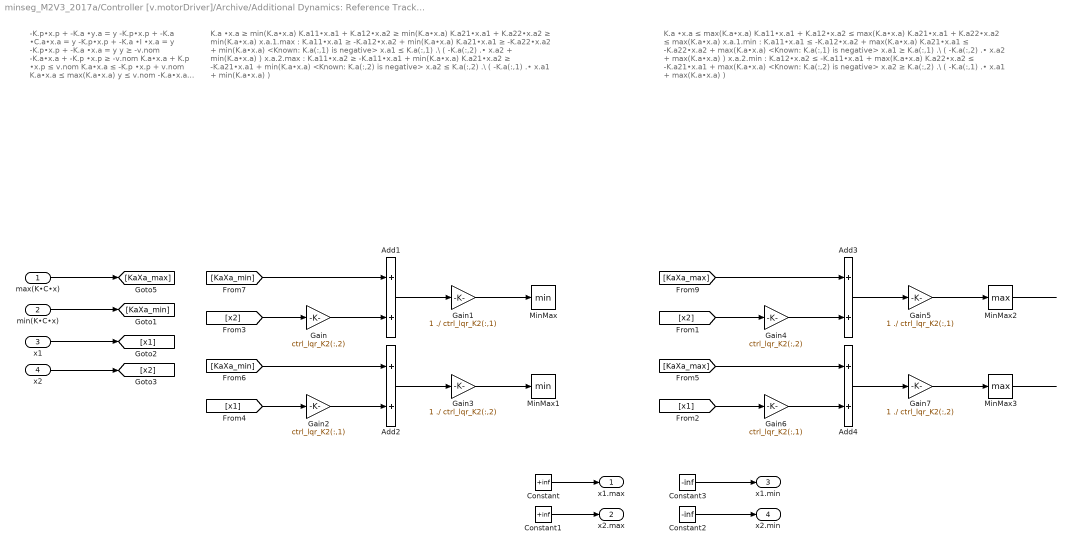
== system minseg_M2V3_2017a/Controller [v.motorDriver]/Archive/Additional Dynamics: Reference Tracking/Delay/Limits Calculation ==
  note: -K.p•x.p + -K.a •y.a = y
      | -K.p•x.p + -K.a •C.a•x.a = y
      | -K.p•x.p + -K.a •I •x.a = y
      | -K.p•x.p + -K.a •x.a = y
      |
      | y ≥ -v.nom
      | -K.a•x.a + -K.p •x.p ≥ -v.nom
      | K.a•x.a + K.p •x.p ≤ v.nom
      | K.a•x.a ≤ -K.p •x.p + v.nom
      | K.a•x.a ≤ max(K.a•x.a)
      |
      | y ≤ v.nom
      | -K.a•x.a + -K.p •x.p ≤ v.nom
      | K.a•x.a + K.p •x.p ≥ -v.nom
      | K.a•x.a ≥ -K.p •x.p + -v.nom
      | K.a•x.a ≥ min(K.a•x.a)
  note: K.a •x.a ≤ max(K.a•x.a)
      |
      | K.a11•x.a1 + K.a12•x.a2 ≤ max(K.a•x.a)
      | K.a21•x.a1 + K.a22•x.a2 ≤ max(K.a•x.a)
      |
      | x.a.1.min :
      |
      | K.a11•x.a1 ≤ -K.a12•x.a2 + max(K.a•x.a)
      | K.a21•x.a1 ≤ -K.a22•x.a2 + max(K.a•x.a)
      |
      | <Known: K.a(:,1) is negative>
      |
      | x.a1 ≥ K.a(:,1) .\ ( -K.a(:,2) .• x.a2 + max(K.a•x.a) )
      |
      | x.a.2.min :
      |
      | K.a12•x.a2 ≤ -K.a11•x.a1 + max(K.a•x.a)
      | K.a22•x.a2 ≤ -K.a21•x.a1 + max(K.a•x.a)
      |
      | <Known: K.a(:,2) is negative>
      |
      | x.a2 ≥ K.a(:,2) .\ ( -K.a(:,1) .• x.a1 + max(K.a•x.a) )
  note: K.a •x.a ≥ min(K.a•x.a)
      |
      | K.a11•x.a1 + K.a12•x.a2 ≥ min(K.a•x.a)
      | K.a21•x.a1 + K.a22•x.a2 ≥ min(K.a•x.a)
      |
      | x.a.1.max :
      |
      | K.a11•x.a1 ≥ -K.a12•x.a2 + min(K.a•x.a)
      | K.a21•x.a1 ≥ -K.a22•x.a2 + min(K.a•x.a)
      |
      | <Known: K.a(:,1) is negative>
      |
      | x.a1 ≤ K.a(:,1) .\ ( -K.a(:,2) .• x.a2 + min(K.a•x.a) )
      |
      | x.a.2.max :
      |
      | K.a11•x.a2 ≥ -K.a11•x.a1 + min(K.a•x.a)
      | K.a21•x.a2 ≥ -K.a21•x.a1 + min(K.a•x.a)
      |
      | <Known: K.a(:,2) is negative>
      |
      | x.a2 ≤ K.a(:,2) .\ ( -K.a(:,1) .• x.a1 + min(K.a•x.a) )
  max(K•C•x) : Inport
  min(K•C•x) : Inport  Port=2
  x1 : Inport  Port=3
  x2 : Inport  Port=4
  Add{1..4} (4 alike) : Sum
  Constant : Constant  Value=+inf  SampleTime=mdl_T_sample
  Constant1 : Constant  Value=+inf  SampleTime=mdl_T_sample
  Constant2 : Constant  Value=-inf  SampleTime=mdl_T_sample
  Constant3 : Constant  Value=-inf  SampleTime=mdl_T_sample
  Gain : Gain  Gain=ctrl_lqr_K2(:,2)
      settings: AttributesFormatString=%<Gain>
  Gain1 : Gain  Gain=1 ./ ctrl_lqr_K2(:,1)
      settings: AttributesFormatString=%<Gain>
  Gain2 : Gain  Gain=ctrl_lqr_K2(:,1)
      settings: AttributesFormatString=%<Gain>
  Gain3 : Gain  Gain=1 ./ ctrl_lqr_K2(:,2)
      settings: AttributesFormatString=%<Gain>
  Gain4 : Gain  Gain=ctrl_lqr_K2(:,2)
      settings: AttributesFormatString=%<Gain>
  Gain5 : Gain  Gain=1 ./ ctrl_lqr_K2(:,1)
      settings: AttributesFormatString=%<Gain>
  Gain6 : Gain  Gain=ctrl_lqr_K2(:,1)
      settings: AttributesFormatString=%<Gain>
  Gain7 : Gain  Gain=1 ./ ctrl_lqr_K2(:,2)
      settings: AttributesFormatString=%<Gain>
  MinMax : MinMax
  MinMax1 : MinMax
  MinMax2 : MinMax  Function=max
  MinMax3 : MinMax  Function=max
  x1.max : Outport
  x2.max : Outport  Port=2
  x1.min : Outport  Port=3
  x2.min : Outport  Port=4
  wires:
  max(K•C•x)/1 -> [KaXa_max]
  min(K•C•x)/1 -> [KaXa_min]
  x1/1 -> [x1]
  x2/1 -> [x2]
  Gain/1 -> Add1/2
  [x2] -> Gain/1
  [KaXa_min] -> Add1/1
  Add1/1 -> Gain1/1
  Gain1/1 -> MinMax/1
  Gain3/1 -> MinMax1/1
  Add2/1 -> Gain3/1
  [x1] -> Gain2/1
  Gain2/1 -> Add2/2
  [KaXa_min] -> Add2/1
  [KaXa_max] -> Add4/1
  Gain6/1 -> Add4/2
  [x1] -> Gain6/1
  Add4/1 -> Gain7/1
  Gain7/1 -> MinMax3/1
  Gain5/1 -> MinMax2/1
  Add3/1 -> Gain5/1
  [KaXa_max] -> Add3/1
  [x2] -> Gain4/1
  Gain4/1 -> Add3/2
  MinMax2/1 -> ?
  MinMax3/1 -> ?
  Constant2/1 -> x2.min/1
  Constant3/1 -> x1.min/1
  Constant1/1 -> x2.max/1
  Constant/1 -> x1.max/1

== system minseg_M2V3_2017a/Controller [v.motorDriver]/Archive/Additional Dynamics: Reference Tracking/Delay/x1 ==
  u.max : Inport
  u[k+1] : Inport  Port=2
  u.min : Inport  Port=3
  reset : Inport  Port=4
  Constant1 : Constant  Value=0  SampleTime=mdl_T_sample
  Saturation flag : Subsystem
  Unit Delay : UnitDelay  InitialCondition=u_init  SampleTime=-1
      settings: AttributesFormatString=initial condition: %<InitialCondition>
  anti-windup : Subsystem
  x.reset : MultiPortSwitch  DataPortOrder=Zero-based contiguous  Inputs=2
  x.saturating : MultiPortSwitch  DataPortOrder=Zero-based contiguous
  u[k] : Outport
  x.sat : Outport  Port=2
  wires:
  [u_kp1] -> Saturation flag/1(u[k+1])
  [u_max] -> Saturation flag/2(u.max)
  [u_min] -> Saturation flag/3(u.min)
  u.min/1 -> [u_min]
  u.max/1 -> [u_max]
  Saturation flag/1(x.saturating) -> [x_sat]
  [x_sat] -> x.sat/1
  [x_sat] -> x.saturating/1
  [u_kp1] -> anti-windup/1(u[k+1].preSat.in), x.saturating/2
  [u_max] -> x.saturating/3
  [u_min] -> x.saturating/4
  u[k+1]/1 -> [u_kp1]
  Constant1/1 -> x.reset/3
  x.reset/1 -> Unit Delay/1
  x.saturating/1 -> anti-windup/2(u[k+1].postSat.in)
  [u] -> u[k]/1
  Unit Delay/1 -> [u]
  anti-windup/1(u[k+1].postSat.out) -> x.reset/2
  reset/1 -> x.reset/1

== system minseg_M2V3_2017a/Controller [v.motorDriver]/Archive/Additional Dynamics: Reference Tracking/Delay/x2 ==
  u.max : Inport
  u[k+1] : Inport  Port=2
  u.min : Inport  Port=3
  reset : Inport  Port=4
  Constant1 : Constant  Value=0  SampleTime=mdl_T_sample
  Saturation flag : Subsystem
  Unit Delay : UnitDelay  InitialCondition=u_init  SampleTime=-1
      settings: AttributesFormatString=initial condition: %<InitialCondition>
  anti-windup : Subsystem
  x.reset : MultiPortSwitch  DataPortOrder=Zero-based contiguous  Inputs=2
  x.saturating : MultiPortSwitch  DataPortOrder=Zero-based contiguous
  u[k] : Outport
  x.sat : Outport  Port=2
  wires:
  reset/1 -> x.reset/1
  anti-windup/1(u[k+1].postSat.out) -> x.reset/2
  Unit Delay/1 -> [u]
  [u] -> u[k]/1
  x.saturating/1 -> anti-windup/2(u[k+1].postSat.in)
  x.reset/1 -> Unit Delay/1
  Constant1/1 -> x.reset/3
  u[k+1]/1 -> [u_kp1]
  [u_min] -> x.saturating/4
  [u_max] -> x.saturating/3
  [u_kp1] -> x.saturating/2, anti-windup/1(u[k+1].preSat.in)
  [x_sat] -> x.saturating/1
  [x_sat] -> x.sat/1
  Saturation flag/1(x.saturating) -> [x_sat]
  u.max/1 -> [u_max]
  u.min/1 -> [u_min]
  [u_min] -> Saturation flag/3(u.min)
  [u_max] -> Saturation flag/2(u.max)
  [u_kp1] -> Saturation flag/1(u[k+1])
